simulink model "Trignomatric_Function"  (R2020a)
settings: Solver=VariableStepAuto  StartTime=0.0  StopTime=10  RelTol=1e-3
settings Model: Creator=Ganesh  LastModifiedBy=Ganesh

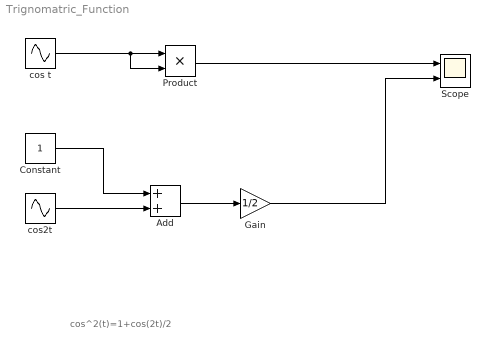
== system Trignomatric_Function ==
  note: cos^2(t)=1+cos(2t)/2
  Add : Sum
  Constant : Constant
  Gain : Gain  Gain=1/2
  Product : Product
  Scope : Scope  NumInputPorts=2
  cos t : Sin  Frequency=2*pi*1  Phase=pi/2  SampleTime=0
  cos2t : Sin  Frequency=2*pi*1*2  Phase=pi/2  SampleTime=0
  wires:
  cos t/1 -> Product/2, Product/1
  Product/1 -> Scope/1
  cos2t/1 -> Add/2
  Constant/1 -> Add/1
  Add/1 -> Gain/1
  Gain/1 -> Scope/2
